simulink model "ICFEMex2"  (R2020a)
settings: Solver=VariableStepAuto  StartTime=0.0  StopTime=10.0  RelTol=1e-3
settings Model: Creator=apple  LastModifiedBy=bzhan
settings DebuggingCC: ArithmeticOperatorsInVariantConditions=warning
settings SFSimCC: CustomCodeUndefinedFunction=UseInterfaceOnly

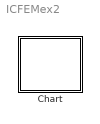
== system ICFEMex2 ==
  Chart : Stateflow chart  TreatAsAtomicUnit=on

== stateflow chart ICFEMex2/Chart ==
  state A
    en: x = 0;
  state B
  A -> (junction 15) [order 1] : [x==0]{fprintf("A");}
  (default) -> A
  A -> B [order 2] : {x=x+1;fprintf("C");}
  data: x local
